simulink model "Plant_2_1"  (R2024b)
settings: Solver=FixedStepAuto  StartTime=0.0  StopTime=20  FixedStep=0.02  RelTol=1e-3
PreLoadFcn:
  | addpath("ref_source\")
model workspace (MAT data in the model file):
  Ref_sig_idx = 2
undefined symbols (not defined in the file or in its folder): A, B, C, D, K, K_r, L1, L2
settings Model: Creator=Sez26  LastModifiedBy=herra

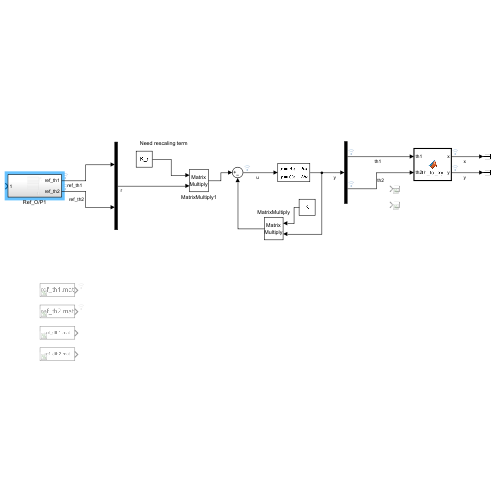
[thumbnail: Simulink's stored preview of the top-level diagram]
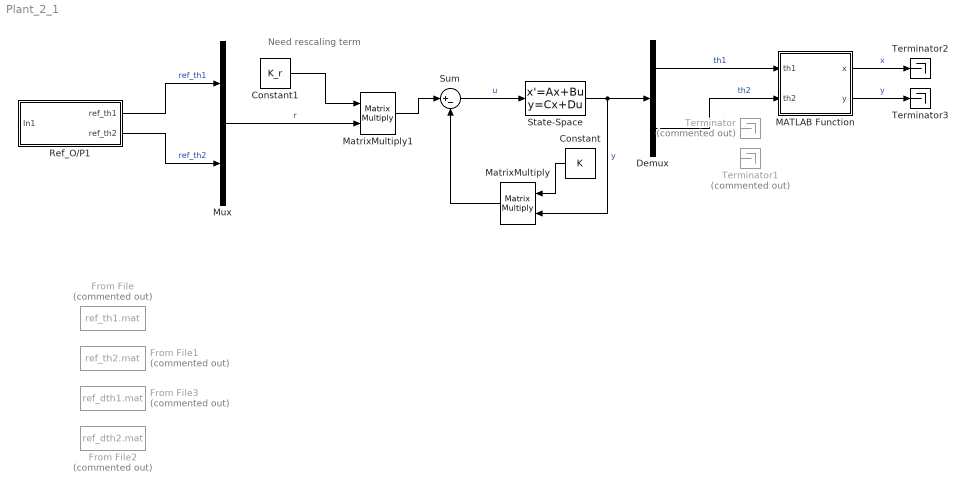
== system Plant_2_1 ==
  note: Need rescaling term
  Constant : Constant  Value=K
  Constant1 : Constant  Value=K_r
  Demux : Demux  Outputs=2
  From File : FromFile  Commented=on  FileName=ref_th1.mat  SampleTime=0
  From File1 : FromFile  Commented=on  FileName=ref_th2.mat  SampleTime=0
  From File2 : FromFile  Commented=on  FileName=ref_dth2.mat  SampleTime=0
  From File3 : FromFile  Commented=on  FileName=ref_dth1.mat  SampleTime=0
  MATLAB Function : MATLAB Function  TreatAsAtomicUnit=on
  MatrixMultiply : Product  Multiplication=Matrix(*)
  MatrixMultiply1 : Product  Multiplication=Matrix(*)
  Mux : Mux  Inputs=2
  Ref_O/P1 : Subsystem
  State-Space : StateSpace  A=A  B=B  C=C  D=D  InitialCondition=0
  Sum : Sum  Inputs=|+-
  Terminator : Terminator  Commented=on
  Terminator1 : Terminator  Commented=on
  Terminator2 : Terminator
  Terminator3 : Terminator
  wires:
  MATLAB Function/1(x) -> Terminator2/1  "x"
  MATLAB Function/2(y) -> Terminator3/1  "y"
  Demux/2 -> MATLAB Function/2(th2)  "th2"
  Demux/1 -> MATLAB Function/1(th1)  "th1"
  Sum/1 -> State-Space/1  "u"
  State-Space/1 -> MatrixMultiply/2, Demux/1  "y"
  MatrixMultiply/1 -> Sum/2
  MatrixMultiply1/1 -> Sum/1
  Mux/1 -> MatrixMultiply1/2  "r"
  Constant1/1 -> MatrixMultiply1/1
  Ref_O/P1/1(ref_th1) -> Mux/1  "ref_th1"
  Ref_O/P1/2(ref_th2) -> Mux/2  "ref_th2"
  Constant/1 -> MatrixMultiply/1

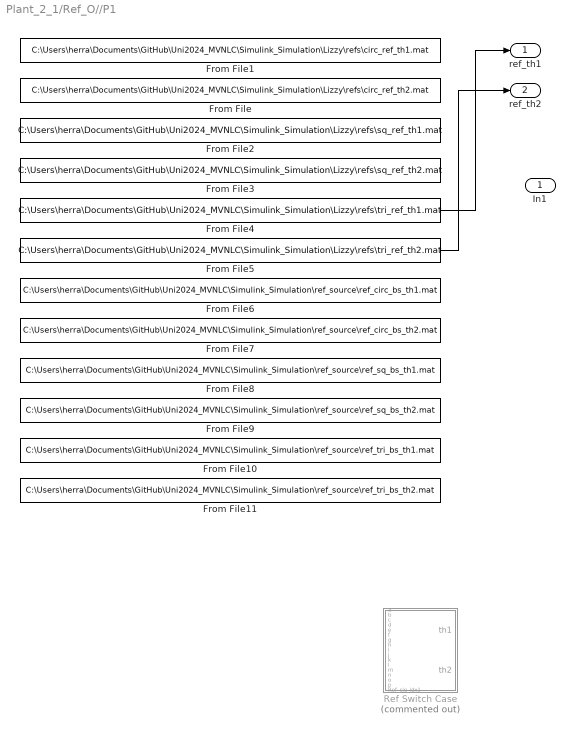
== system Plant_2_1/Ref_O//P1 ==
  In1 : Inport
  From File : FromFile  FileName=C:\Users\herra\Documents\GitHub\Uni2024_MVNLC\Simulink_Simulation\Lizzy\refs\circ_ref_th2.mat  SampleTime=0
  From File1 : FromFile  FileName=C:\Users\herra\Documents\GitHub\Uni2024_MVNLC\Simulink_Simulation\Lizzy\refs\circ_ref_th1.mat  SampleTime=0
  From File10 : FromFile  FileName=C:\Users\herra\Documents\GitHub\Uni2024_MVNLC\Simulink_Simulation\ref_source\ref_tri_bs_th1.mat  SampleTime=0
  From File11 : FromFile  FileName=C:\Users\herra\Documents\GitHub\Uni2024_MVNLC\Simulink_Simulation\ref_source\ref_tri_bs_th2.mat  SampleTime=0
  From File2 : FromFile  FileName=C:\Users\herra\Documents\GitHub\Uni2024_MVNLC\Simulink_Simulation\Lizzy\refs\sq_ref_th1.mat  SampleTime=0
  From File3 : FromFile  FileName=C:\Users\herra\Documents\GitHub\Uni2024_MVNLC\Simulink_Simulation\Lizzy\refs\sq_ref_th2.mat  SampleTime=0
  From File4 : FromFile  FileName=C:\Users\herra\Documents\GitHub\Uni2024_MVNLC\Simulink_Simulation\Lizzy\refs\tri_ref_th1.mat  SampleTime=0
  From File5 : FromFile  FileName=C:\Users\herra\Documents\GitHub\Uni2024_MVNLC\Simulink_Simulation\Lizzy\refs\tri_ref_th2.mat  SampleTime=0
  From File6 : FromFile  FileName=C:\Users\herra\Documents\GitHub\Uni2024_MVNLC\Simulink_Simulation\ref_source\ref_circ_bs_th1.mat  SampleTime=0
  From File7 : FromFile  FileName=C:\Users\herra\Documents\GitHub\Uni2024_MVNLC\Simulink_Simulation\ref_source\ref_circ_bs_th2.mat  SampleTime=0
  From File8 : FromFile  FileName=C:\Users\herra\Documents\GitHub\Uni2024_MVNLC\Simulink_Simulation\ref_source\ref_sq_bs_th1.mat  SampleTime=0
  From File9 : FromFile  FileName=C:\Users\herra\Documents\GitHub\Uni2024_MVNLC\Simulink_Simulation\ref_source\ref_sq_bs_th2.mat  SampleTime=0
  Ref Switch Case : MATLAB Function  Commented=on  TreatAsAtomicUnit=on
  ref_th1 : Outport
  ref_th2 : Outport  Port=2
  wires:
  From File4/1 -> ref_th1/1
  From File5/1 -> ref_th2/1

== matlab function Plant_2_1/MATLAB Function ==
  data: x output; th1 input; y output; th2 input; L1 parameter; L2 parameter
function [x,y] = th_to_xy(th1, th2, L1, L2)
    x = L1*cos(deg2rad(th1)) + L2*cos(deg2rad(th2));
    y = L1*sin(deg2rad(th1)) + L2*sin(deg2rad(th2));

== matlab function Plant_2_1/Ref_O//P1/Ref Switch Case ==
  data: Ref_sig_idx parameter; a input; b input; c input; d input; e input; f input; g input; h input; i input; j input; k input; l input; m input; n input; o input; p input; Ref_sig_idx1 input; th1 output; th2 output
function [th1, th2] = ref_switch(Ref_sig_idx, a, b, c, d, e, f, g, h, i, j, k, l, m, n, o, p, Ref_sig_idx1)
    if Ref_sig_idx == 0
        % circ base
        th1 = a;
        th2 = b;
    elseif Ref_sig_idx == 1
        % sq base
        th1 = c;
        th2 = d;
    elseif Ref_sig_idx == 2
        % tri base
        th1 = e;
        th2 = f;
    end
    if Ref_sig_idx == 3
        % circ b spline
        th1 = g;
        th2 = h;
    elseif Ref_sig_idx == 4
        % sq b spline
        th1 = i;
        th2 = j;
    elseif Ref_sig_idx == 5
        % tri b spline
        th1 = k;
        th2 = l;
    end
    if Ref_sig_idx == 6
        % sq corner sf
        th1 = m;
        th2 = n;
    elseif Ref_sig_idx == 7
        % tri corner sf
        th1 = o;
        th2 = p;
    else
        % invalid reference choice
        disp('Error invalid reference choice')
        th1 = 0;
        th2 = 0;
    end
